simulink model "sim_3"  (R2021a)
settings: Solver=ode4  StartTime=0.0  StopTime=10.0  FixedStep=0.001  RelTol=1e-3
libraries: cstblocks x4
settings Model: Creator=me-clab2  LastModifiedBy=HASEE
settings SolverCC: AlgebraicLoopSolver=TrustRegion
settings DebuggingCC: SFMachineParentedDataDiag=warning

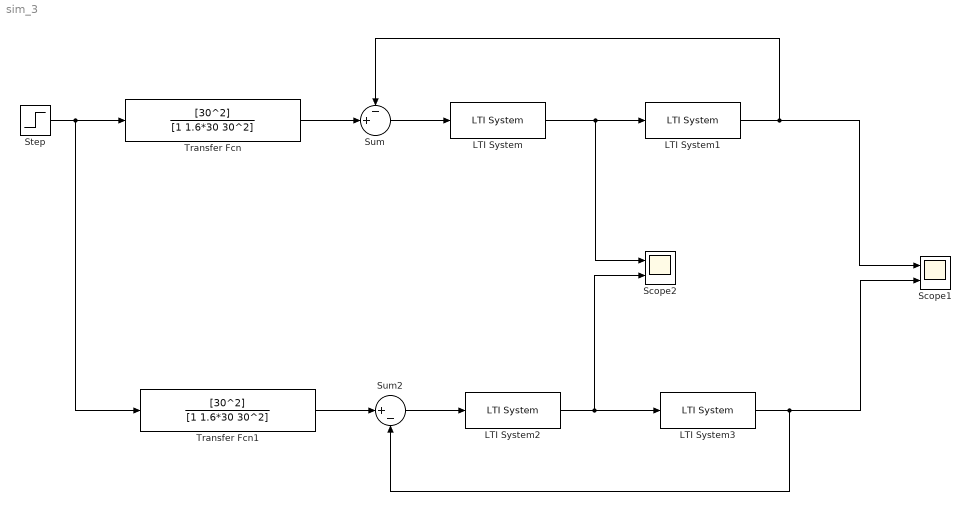
== system sim_3 ==
  LTI System : cstblocks/LTI System  sys=C2  IC=[]
  LTI System1 : cstblocks/LTI System  sys=P  IC=[]
  LTI System2 : cstblocks/LTI System  sys=C3  IC=[]
  LTI System3 : cstblocks/LTI System  sys=P  IC=[]
  Scope1 : Scope  NumInputPorts=2
  Scope2 : Scope  NumInputPorts=2
  Step : Step  Time=0  After=30  SampleTime=0
  Sum : Sum  Inputs=-+|
  Sum2 : Sum  Inputs=|+-
  Transfer Fcn : TransferFcn  Numerator=[30^2]  Denominator=[1 1.6*30 30^2]
  Transfer Fcn1 : TransferFcn  Numerator=[30^2]  Denominator=[1 1.6*30 30^2]
  wires:
  Sum/1 -> LTI System/1
  LTI System1/1 -> Scope1/1, Sum/1
  Step/1 -> Transfer Fcn1/1, Transfer Fcn/1
  Sum2/1 -> LTI System2/1
  LTI System3/1 -> Scope1/2, Sum2/2
  Transfer Fcn1/1 -> Sum2/1
  LTI System/1 -> Scope2/1, LTI System1/1
  LTI System2/1 -> Scope2/2, LTI System3/1
  Transfer Fcn/1 -> Sum/2
